simulink model "Robust_joint_Space_DIST"  (R2020b)
settings: Solver=VariableStepAuto  StartTime=0.0  StopTime=50  RelTol=1e-3
libraries: simulink x1
(part 1 of 4)
settings Model: Creator=Asus  LastModifiedBy=Asus

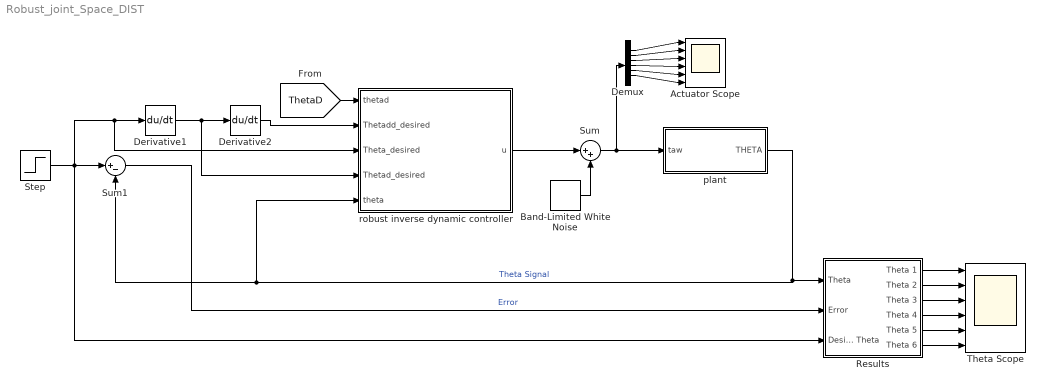
== system Robust_joint_Space_DIST ==
  Actuator Scope : Scope  NumInputPorts=6
  Band-Limited White Noise : simulink/Sources/Band-Limited White Noise  Cov=[0.001]  Ts=0.1  seed=[23341]
  Demux : Demux  Outputs=6
  Derivative1 : Derivative
  Derivative2 : Derivative
  Results : Subsystem
  Step : Step  Time=0  Before=[0;0;0;0;0;0];  After=[pi/2;pi/2;pi/2;pi/2;pi/2;pi/2];  SampleTime=0
  Sum : Sum  Inputs=|++
  Sum1 : Sum  Inputs=|+-
  Theta Scope : Scope  NumInputPorts=6
  plant : Subsystem
  robust inverse dynamic controller : Subsystem
  wires:
  Step/1 -> Results/3(Desired Theta), Derivative1/1, robust inverse dynamic controller/3(Theta_desired), Sum1/1
  [ThetaD] -> robust inverse dynamic controller/1(thetad)
  Demux/5 -> Actuator Scope/5
  Results/4(Theta 4) -> Theta Scope/4
  Results/1(Theta 1) -> Theta Scope/1
  Results/5(Theta 5) -> Theta Scope/5
  Demux/4 -> Actuator Scope/4
  Demux/6 -> Actuator Scope/6
  Results/6(Theta 6) -> Theta Scope/6
  Results/3(Theta 3) -> Theta Scope/3
  Demux/3 -> Actuator Scope/3
  Demux/2 -> Actuator Scope/2
  Derivative2/1 -> robust inverse dynamic controller/2(Thetadd_desired)
  Demux/1 -> Actuator Scope/1
  plant/1(THETA) -> Sum1/2, robust inverse dynamic controller/5(theta), Results/1(Theta)  "Theta Signal"
  Derivative1/1 -> robust inverse dynamic controller/4(Thetad_desired), Derivative2/1
  Results/2(Theta 2) -> Theta Scope/2
  Sum1/1 -> Results/2(Error)  "Error"
  Band-Limited White Noise/1 -> Sum/2
  robust inverse dynamic controller/1(u) -> Sum/1
  Sum/1 -> Demux/1, plant/1(taw)

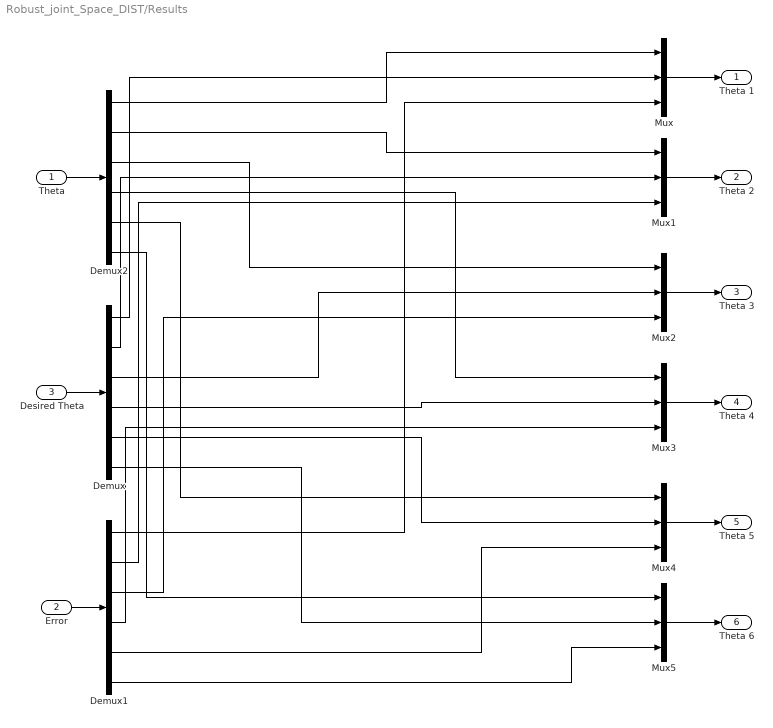
== system Robust_joint_Space_DIST/Results ==
  Theta : Inport
  Error : Inport  Port=2
  Desired Theta : Inport  Port=3
  Demux : Demux  Outputs=6
  Demux1 : Demux  Outputs=6
  Demux2 : Demux  Outputs=6
  Mux{,1..5} (6 alike) : Mux  Inputs=3
  Theta 1 : Outport  VectorParamsAs1DForOutWhenUnconnected=off
  Theta 2 : Outport  Port=2  VectorParamsAs1DForOutWhenUnconnected=off
  Theta 3 : Outport  Port=3  VectorParamsAs1DForOutWhenUnconnected=off
  Theta 4 : Outport  Port=4  VectorParamsAs1DForOutWhenUnconnected=off
  Theta 5 : Outport  Port=5  VectorParamsAs1DForOutWhenUnconnected=off
  Theta 6 : Outport  Port=6  VectorParamsAs1DForOutWhenUnconnected=off
  wires:
  Desired Theta/1 -> Demux/1
  Error/1 -> Demux1/1
  Theta/1 -> Demux2/1
  Mux/1 -> Theta 1/1
  Mux1/1 -> Theta 2/1
  Mux2/1 -> Theta 3/1
  Mux3/1 -> Theta 4/1
  Mux4/1 -> Theta 5/1
  Mux5/1 -> Theta 6/1
  Demux2/1 -> Mux/1
  Demux2/2 -> Mux1/1
  Demux2/3 -> Mux2/1
  Demux2/4 -> Mux3/1
  Demux2/5 -> Mux4/1
  Demux2/6 -> Mux5/1
  Demux/1 -> Mux/2
  Demux/2 -> Mux1/2
  Demux/3 -> Mux2/2
  Demux/4 -> Mux3/2
  Demux/5 -> Mux4/2
  Demux/6 -> Mux5/2
  Demux1/1 -> Mux/3
  Demux1/2 -> Mux1/3
  Demux1/3 -> Mux2/3
  Demux1/4 -> Mux3/3
  Demux1/5 -> Mux4/3
  Demux1/6 -> Mux5/3

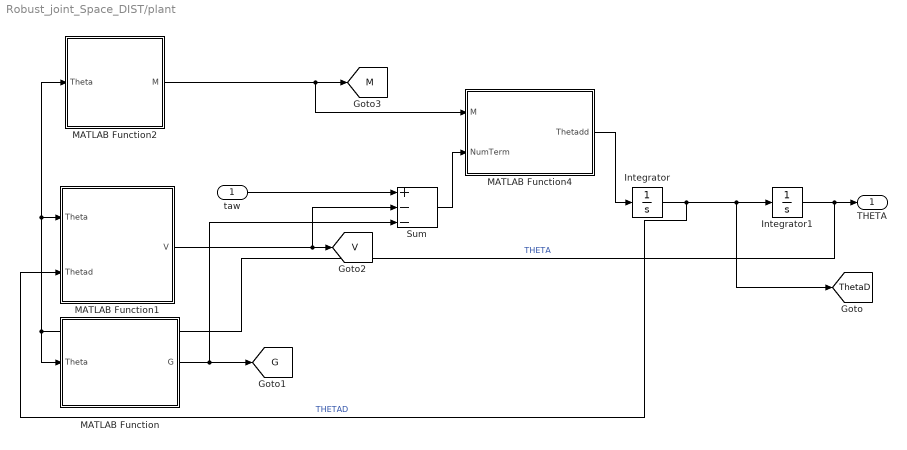
== system Robust_joint_Space_DIST/plant ==
  taw : Inport
  Integrator : Integrator  InitialCondition=[0;0;0;0;0;0]
  Integrator1 : Integrator  InitialCondition=[0;0;0;0;0;0]
  MATLAB Function : MATLAB Function  TreatAsAtomicUnit=on
  MATLAB Function1 : MATLAB Function  TreatAsAtomicUnit=on
  MATLAB Function2 : MATLAB Function  TreatAsAtomicUnit=on
  MATLAB Function4 : MATLAB Function  TreatAsAtomicUnit=on
  Sum : Sum  Inputs=+--
  THETA : Outport
  tag scope: G=global, M=global, ThetaD=global, V=global
  wires:
  Integrator/1 -> MATLAB Function1/2(Thetad), [ThetaD], Integrator1/1  "THETAD"
  MATLAB Function4/1(Thetadd) -> Integrator/1
  MATLAB Function1/1(V) -> Sum/2, [V]
  MATLAB Function2/1(M) -> [M], MATLAB Function4/1(M)
  Sum/1 -> MATLAB Function4/2(NumTerm)
  Integrator1/1 -> MATLAB Function1/1(Theta), MATLAB Function2/1(Theta), MATLAB Function/1(Theta), THETA/1  "THETA"
  taw/1 -> Sum/1
  MATLAB Function/1(G) -> Sum/3, [G]

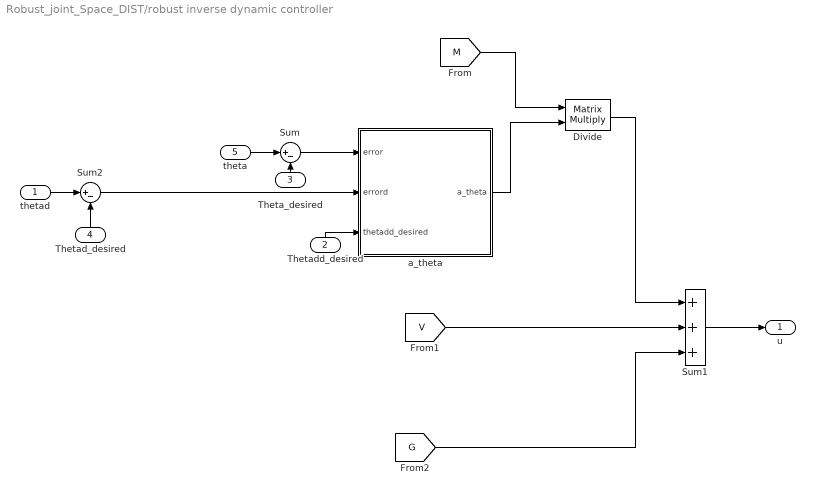
== system Robust_joint_Space_DIST/robust inverse dynamic controller ==
  thetad : Inport
  Thetadd_desired : Inport  Port=2
  Theta_desired : Inport  Port=3
  Thetad_desired : Inport  Port=4
  theta : Inport  Port=5
  Divide : Product  Multiplication=Matrix(*)
  Sum : Sum  Inputs=|+-
  Sum1 : Sum  Inputs=+++
  Sum2 : Sum  Inputs=|+-
  a_theta : MATLAB Function  TreatAsAtomicUnit=on
  u : Outport
  wires:
  a_theta/1(a_theta) -> Divide/2
  Sum1/1 -> u/1
  [G] -> Sum1/3
  Divide/1 -> Sum1/1
  [V] -> Sum1/2
  theta/1 -> Sum/1
  thetad/1 -> Sum2/1
  Thetadd_desired/1 -> a_theta/3(thetadd_desired)
  Thetad_desired/1 -> Sum2/2
  Sum2/1 -> a_theta/2(errord)
  Theta_desired/1 -> Sum/2
  Sum/1 -> a_theta/1(error)
  [M] -> Divide/1
